simulink model "ControlSystem"  (R2021b)
settings: Solver=VariableStepAuto  StartTime=simIn(1,1)  StopTime=simIn(end,1)  RelTol=1e-3
values from neighbouring files (symbols this model uses):
  A = -inv(L)*R    [PlasmalessModel.m]
  B = L\S    [PlasmalessModel.m]
  C = eye(circuitNumber,length(A))    [PlasmalessModel.m]
  Controller = struct('R1',pid(Rcontr(1,1)),'R2',pid(Rcontr(2,2)),'R3',pid(Rcontr(3,3)),'R4',pid(Rcontr(4,4)),'R5',      pid(Rcontr(5,5)),'R6',pid(Rcontr(6,6)),'R7',pid(Rcontr(7,7)),'R8',pid(Rcontr(8,8)),'R9',pid(Rcontr(9,9)),'R10',      pid(Rcontr(10,10)),'R11',pid(Rcontr(11,11)),'R12',pid(Rcontr(12,12)))    [GeneticAlgorithm.m]    (also in OptimalTunedGA.mat = ; PIDController.m = struct('R1',R1,'R2',R2,'R3',R3,'R4',R4,'R5',R5,'R6',R6,     ; RLocusController.m = struct('R1',R1,'R2',R2,'R3',R3,'R4',R4,'R5',R5,'R6',R6,     )
  D = zeros(circuitNumber,circuitNumber)    [PlasmalessModel.m]
  dt = 0.001    [GeneticAlgorithm.m]    (also in PlasmalessModel.m; ReferenceDatabase.m)
  fil1 = zpk(minreal(R1 - k1 - r1(end)/s, 1e-2))    [RLocusController.m]
  fil10 = zpk(minreal(R10 - k10 - r10(end)/s, 1e-2))    [RLocusController.m]
  fil11 = zpk(minreal(R11 - k11 - r11(end)/s, 1e-2))    [RLocusController.m]
  fil12 = zpk(minreal(R12 - k12 - r12(end)/s, 1e-2))    [RLocusController.m]
  fil2 = zpk(minreal(R2 - k2 - r2(end)/s, 1e-2))    [RLocusController.m]
  fil3 = zpk(minreal(R3 - k3 - r3(end)/s, 1e-2))    [RLocusController.m]
  fil4 = zpk(minreal(R4 - k4 - r4(end)/s, 1e-2))    [RLocusController.m]
  fil5 = zpk(minreal(R5 - k5 - r5(end)/s, 1e-2))    [RLocusController.m]
  fil6 = zpk(minreal(R6 - k6 - r6(end)/s, 1e-2))    [RLocusController.m]
  fil7 = zpk(minreal(R7 - k7 - r7(end)/s, 1e-2))    [RLocusController.m]
  fil8 = zpk(minreal(R8 - k8 - r8(end)/s, 1e-2))    [RLocusController.m]
  fil9 = zpk(minreal(R9 - k9 - r9(end)/s, 1e-2))    [RLocusController.m]
  PSdelay = 1.67e-3    (= 0.00167)    [PlasmalessModel.m]
  PSden = [7e-3 1]    [PlasmalessModel.m]
  PSnum = 1    [PlasmalessModel.m]
  PSsat = [350 350 350 350 350 350           800 800 400 400 330 330]    [PlasmalessModel.m]
  sys1 = balred(sys(1,1),ord)    [PlasmalessModel.m]
  sys10 = balred(sys(10,10),ord)    [PlasmalessModel.m]
  sys11 = balred(sys(11,11),ord)    [PlasmalessModel.m]
  sys12 = balred(sys(12,12),ord)    [PlasmalessModel.m]
  sys2 = balred(sys(2,2),ord)    [PlasmalessModel.m]
  sys3 = balred(sys(3,3),ord)    [PlasmalessModel.m]
  sys4 = balred(sys(4,4),ord)    [PlasmalessModel.m]
  sys5 = balred(sys(5,5),ord)    [PlasmalessModel.m]
  sys6 = balred(sys(6,6),ord)    [PlasmalessModel.m]
  sys7 = balred(sys(7,7),ord)    [PlasmalessModel.m]
  sys8 = balred(sys(8,8),ord)    [PlasmalessModel.m]
  sys9 = balred(sys(9,9),ord)    [PlasmalessModel.m]
  varIpf = Scenario.Reference4.var    [PlasmalessModel.m]    (also in ReferenceDatabase.m)
undefined symbols (not defined in the file or in its folder): k1, k10, k11, k12, k2, k3, k4, k5, k6, k7, k8, k9
libraries: simulink x98, cstblocks x60
(part 3 of 4)

== system ControlSystem/Variant system/SISO/Variant Controller/PID/Subsystem13 ==
  e : Inport
  antiw : Inport  Port=2
  Avoid windup : Constant  Value=0
  Clamping : Subsystem
  Derivative Gain : Gain  Gain=Kd
  Filtered Derivative : TransferFcn  Denominator=Tf
  Integral Gain : Gain  Gain=Ki
  Integrator : Integrator
  Proportional Gain : Gain  Gain=Kp
  Sum action : Sum  Inputs=+++
  Switch1 : Switch  Criteria=u2 > Threshold
  u : Outport
  wires:
  Filtered Derivative/1 -> Sum action/2
  Sum action/1 -> Clamping/1(u), u/1  "u"
  Derivative Gain/1 -> Filtered Derivative/1
  e/1 -> Proportional Gain/1, Clamping/3(e), Integral Gain/1, Derivative Gain/1  "e"
  Switch1/1 -> Integrator/1
  Integral Gain/1 -> Switch1/3
  Avoid windup/1 -> Switch1/1
  Proportional Gain/1 -> Sum action/1
  Integrator/1 -> Sum action/3
  antiw/1 -> Clamping/2(antiw)  "antiw"
  Clamping/1(Clamping) -> Switch1/2  "Clamping"

== system ControlSystem/Variant system/SISO/Variant Controller/PID/Subsystem2 ==
  e : Inport
  antiw : Inport  Port=2
  Avoid windup : Constant  Value=0
  Clamping : Subsystem
  Derivative Gain : Gain  Gain=Kd
  Filtered Derivative : TransferFcn  Denominator=Tf
  Integral Gain : Gain  Gain=Ki
  Integrator : Integrator
  Proportional Gain : Gain  Gain=Kp
  Sum action : Sum  Inputs=+++
  Switch1 : Switch  Criteria=u2 > Threshold
  u : Outport
  wires:
  Clamping/1(Clamping) -> Switch1/2  "Clamping"
  antiw/1 -> Clamping/2(antiw)  "antiw"
  Integrator/1 -> Sum action/3
  Proportional Gain/1 -> Sum action/1
  Avoid windup/1 -> Switch1/1
  Integral Gain/1 -> Switch1/3
  Switch1/1 -> Integrator/1
  e/1 -> Derivative Gain/1, Integral Gain/1, Clamping/3(e), Proportional Gain/1  "e"
  Derivative Gain/1 -> Filtered Derivative/1
  Sum action/1 -> u/1, Clamping/1(u)  "u"
  Filtered Derivative/1 -> Sum action/2

== system ControlSystem/Variant system/SISO/Variant Controller/PID/Subsystem3 ==
  e : Inport
  antiw : Inport  Port=2
  Avoid windup : Constant  Value=0
  Clamping : Subsystem
  Derivative Gain : Gain  Gain=Kd
  Filtered Derivative : TransferFcn  Denominator=Tf
  Integral Gain : Gain  Gain=Ki
  Integrator : Integrator
  Proportional Gain : Gain  Gain=Kp
  Sum action : Sum  Inputs=+++
  Switch1 : Switch  Criteria=u2 > Threshold
  u : Outport
  wires:
  Filtered Derivative/1 -> Sum action/2
  Sum action/1 -> Clamping/1(u), u/1  "u"
  Derivative Gain/1 -> Filtered Derivative/1
  e/1 -> Proportional Gain/1, Clamping/3(e), Integral Gain/1, Derivative Gain/1  "e"
  Switch1/1 -> Integrator/1
  Integral Gain/1 -> Switch1/3
  Avoid windup/1 -> Switch1/1
  Proportional Gain/1 -> Sum action/1
  Integrator/1 -> Sum action/3
  antiw/1 -> Clamping/2(antiw)  "antiw"
  Clamping/1(Clamping) -> Switch1/2  "Clamping"

== system ControlSystem/Variant system/SISO/Variant Controller/PID/Subsystem4 ==
  e : Inport
  antiw : Inport  Port=2
  Avoid windup : Constant  Value=0
  Clamping : Subsystem
  Derivative Gain : Gain  Gain=Kd
  Filtered Derivative : TransferFcn  Denominator=Tf
  Integral Gain : Gain  Gain=Ki
  Integrator : Integrator
  Proportional Gain : Gain  Gain=Kp
  Sum action : Sum  Inputs=+++
  Switch1 : Switch  Criteria=u2 > Threshold
  u : Outport
  wires:
  Clamping/1(Clamping) -> Switch1/2  "Clamping"
  antiw/1 -> Clamping/2(antiw)  "antiw"
  Integrator/1 -> Sum action/3
  Proportional Gain/1 -> Sum action/1
  Avoid windup/1 -> Switch1/1
  Integral Gain/1 -> Switch1/3
  Switch1/1 -> Integrator/1
  e/1 -> Derivative Gain/1, Integral Gain/1, Clamping/3(e), Proportional Gain/1  "e"
  Derivative Gain/1 -> Filtered Derivative/1
  Sum action/1 -> u/1, Clamping/1(u)  "u"
  Filtered Derivative/1 -> Sum action/2

== system ControlSystem/Variant system/SISO/Variant Controller/PID/Subsystem5 ==
  e : Inport
  antiw : Inport  Port=2
  Avoid windup : Constant  Value=0
  Clamping : Subsystem
  Derivative Gain : Gain  Gain=Kd
  Filtered Derivative : TransferFcn  Denominator=Tf
  Integral Gain : Gain  Gain=Ki
  Integrator : Integrator
  Proportional Gain : Gain  Gain=Kp
  Sum action : Sum  Inputs=+++
  Switch1 : Switch  Criteria=u2 > Threshold
  u : Outport
  wires:
  Filtered Derivative/1 -> Sum action/2
  Sum action/1 -> Clamping/1(u), u/1  "u"
  Derivative Gain/1 -> Filtered Derivative/1
  e/1 -> Proportional Gain/1, Clamping/3(e), Integral Gain/1, Derivative Gain/1  "e"
  Switch1/1 -> Integrator/1
  Integral Gain/1 -> Switch1/3
  Avoid windup/1 -> Switch1/1
  Proportional Gain/1 -> Sum action/1
  Integrator/1 -> Sum action/3
  antiw/1 -> Clamping/2(antiw)  "antiw"
  Clamping/1(Clamping) -> Switch1/2  "Clamping"

== system ControlSystem/Variant system/SISO/Variant Controller/PID/Subsystem6 ==
  e : Inport
  antiw : Inport  Port=2
  Avoid windup : Constant  Value=0
  Clamping : Subsystem
  Derivative Gain : Gain  Gain=Kd
  Filtered Derivative : TransferFcn  Denominator=Tf
  Integral Gain : Gain  Gain=Ki
  Integrator : Integrator
  Proportional Gain : Gain  Gain=Kp
  Sum action : Sum  Inputs=+++
  Switch1 : Switch  Criteria=u2 > Threshold
  u : Outport
  wires:
  Clamping/1(Clamping) -> Switch1/2  "Clamping"
  antiw/1 -> Clamping/2(antiw)  "antiw"
  Integrator/1 -> Sum action/3
  Proportional Gain/1 -> Sum action/1
  Avoid windup/1 -> Switch1/1
  Integral Gain/1 -> Switch1/3
  Switch1/1 -> Integrator/1
  e/1 -> Derivative Gain/1, Integral Gain/1, Clamping/3(e), Proportional Gain/1  "e"
  Derivative Gain/1 -> Filtered Derivative/1
  Sum action/1 -> u/1, Clamping/1(u)  "u"
  Filtered Derivative/1 -> Sum action/2

== system ControlSystem/Variant system/SISO/Variant Controller/PID/Subsystem7 ==
  e : Inport
  antiw : Inport  Port=2
  Avoid windup : Constant  Value=0
  Clamping : Subsystem
  Derivative Gain : Gain  Gain=Kd
  Filtered Derivative : TransferFcn  Denominator=Tf
  Integral Gain : Gain  Gain=Ki
  Integrator : Integrator
  Proportional Gain : Gain  Gain=Kp
  Sum action : Sum  Inputs=+++
  Switch1 : Switch  Criteria=u2 > Threshold
  u : Outport
  wires:
  Filtered Derivative/1 -> Sum action/2
  Sum action/1 -> Clamping/1(u), u/1  "u"
  Derivative Gain/1 -> Filtered Derivative/1
  e/1 -> Proportional Gain/1, Clamping/3(e), Integral Gain/1, Derivative Gain/1  "e"
  Switch1/1 -> Integrator/1
  Integral Gain/1 -> Switch1/3
  Avoid windup/1 -> Switch1/1
  Proportional Gain/1 -> Sum action/1
  Integrator/1 -> Sum action/3
  antiw/1 -> Clamping/2(antiw)  "antiw"
  Clamping/1(Clamping) -> Switch1/2  "Clamping"

== system ControlSystem/Variant system/SISO/Variant Controller/PID/Subsystem8 ==
  e : Inport
  antiw : Inport  Port=2
  Avoid windup : Constant  Value=0
  Clamping : Subsystem
  Derivative Gain : Gain  Gain=Kd
  Filtered Derivative : TransferFcn  Denominator=Tf
  Integral Gain : Gain  Gain=Ki
  Integrator : Integrator
  Proportional Gain : Gain  Gain=Kp
  Sum action : Sum  Inputs=+++
  Switch1 : Switch  Criteria=u2 > Threshold
  u : Outport
  wires:
  Clamping/1(Clamping) -> Switch1/2  "Clamping"
  antiw/1 -> Clamping/2(antiw)  "antiw"
  Integrator/1 -> Sum action/3
  Proportional Gain/1 -> Sum action/1
  Avoid windup/1 -> Switch1/1
  Integral Gain/1 -> Switch1/3
  Switch1/1 -> Integrator/1
  e/1 -> Derivative Gain/1, Integral Gain/1, Clamping/3(e), Proportional Gain/1  "e"
  Derivative Gain/1 -> Filtered Derivative/1
  Sum action/1 -> u/1, Clamping/1(u)  "u"
  Filtered Derivative/1 -> Sum action/2

== system ControlSystem/Variant system/SISO/Variant Controller/PID/Subsystem9 ==
  e : Inport
  antiw : Inport  Port=2
  Avoid windup : Constant  Value=0
  Clamping : Subsystem
  Derivative Gain : Gain  Gain=Kd
  Filtered Derivative : TransferFcn  Denominator=Tf
  Integral Gain : Gain  Gain=Ki
  Integrator : Integrator
  Proportional Gain : Gain  Gain=Kp
  Sum action : Sum  Inputs=+++
  Switch1 : Switch  Criteria=u2 > Threshold
  u : Outport
  wires:
  Filtered Derivative/1 -> Sum action/2
  Sum action/1 -> Clamping/1(u), u/1  "u"
  Derivative Gain/1 -> Filtered Derivative/1
  e/1 -> Proportional Gain/1, Clamping/3(e), Integral Gain/1, Derivative Gain/1  "e"
  Switch1/1 -> Integrator/1
  Integral Gain/1 -> Switch1/3
  Avoid windup/1 -> Switch1/1
  Proportional Gain/1 -> Sum action/1
  Integrator/1 -> Sum action/3
  antiw/1 -> Clamping/2(antiw)  "antiw"
  Clamping/1(Clamping) -> Switch1/2  "Clamping"

== system ControlSystem/Variant system/SISO/Variant Controller/Rlocusantiwindup/Subsystem1 ==
  e : Inport
  antiw : Inport  Port=2
  Avoid windup : Constant  Value=0
  Clamping : Subsystem
  Integral Gain : Gain  Gain=Ki
  Integrator : Integrator
  Proportional Gain : Gain  Gain=Kp
  Sum action : Sum  Inputs=+++
  Switch1 : Switch  Criteria=u2 > Threshold
  ZPK compensator : cstblocks/LTI System  sys=Compensator  IC=[]
  u : Outport
  wires:
  Sum action/1 -> Clamping/1(u), u/1  "u"
  ZPK compensator/1 -> Sum action/2
  e/1 -> ZPK compensator/1, Proportional Gain/1, Clamping/3(e), Integral Gain/1  "e"
  Switch1/1 -> Integrator/1
  Integral Gain/1 -> Switch1/3
  Avoid windup/1 -> Switch1/1
  Proportional Gain/1 -> Sum action/1
  Integrator/1 -> Sum action/3
  antiw/1 -> Clamping/2(antiw)  "antiw"
  Clamping/1(Clamping) -> Switch1/2  "Clamping"

== system ControlSystem/Variant system/SISO/Variant Controller/Rlocusantiwindup/Subsystem11 ==
  e : Inport
  antiw : Inport  Port=2
  Avoid windup : Constant  Value=0
  Clamping : Subsystem
  Integral Gain : Gain  Gain=Ki
  Integrator : Integrator
  Proportional Gain : Gain  Gain=Kp
  Sum action : Sum  Inputs=+++
  Switch1 : Switch  Criteria=u2 > Threshold
  ZPK compensator : cstblocks/LTI System  sys=Compensator  IC=[]
  u : Outport
  wires:
  Clamping/1(Clamping) -> Switch1/2  "Clamping"
  antiw/1 -> Clamping/2(antiw)  "antiw"
  Integrator/1 -> Sum action/3
  Proportional Gain/1 -> Sum action/1
  Avoid windup/1 -> Switch1/1
  Integral Gain/1 -> Switch1/3
  Switch1/1 -> Integrator/1
  e/1 -> Integral Gain/1, Clamping/3(e), Proportional Gain/1, ZPK compensator/1  "e"
  ZPK compensator/1 -> Sum action/2
  Sum action/1 -> u/1, Clamping/1(u)  "u"

== system ControlSystem/Variant system/SISO/Variant Controller/Rlocusantiwindup/Subsystem12 ==
  e : Inport
  antiw : Inport  Port=2
  Avoid windup : Constant  Value=0
  Clamping : Subsystem
  Integral Gain : Gain  Gain=Ki
  Integrator : Integrator
  Proportional Gain : Gain  Gain=Kp
  Sum action : Sum  Inputs=+++
  Switch1 : Switch  Criteria=u2 > Threshold
  ZPK compensator : cstblocks/LTI System  sys=Compensator  IC=[]
  u : Outport
  wires:
  Clamping/1(Clamping) -> Switch1/2  "Clamping"
  antiw/1 -> Clamping/2(antiw)  "antiw"
  Integrator/1 -> Sum action/3
  Proportional Gain/1 -> Sum action/1
  Avoid windup/1 -> Switch1/1
  Integral Gain/1 -> Switch1/3
  Switch1/1 -> Integrator/1
  e/1 -> Integral Gain/1, Clamping/3(e), Proportional Gain/1, ZPK compensator/1  "e"
  ZPK compensator/1 -> Sum action/2
  Sum action/1 -> u/1, Clamping/1(u)  "u"

== system ControlSystem/Variant system/SISO/Variant Controller/Rlocusantiwindup/Subsystem15 ==
  e : Inport
  antiw : Inport  Port=2
  Avoid windup : Constant  Value=0
  Clamping : Subsystem
  Integral Gain : Gain  Gain=Ki
  Integrator : Integrator
  Proportional Gain : Gain  Gain=Kp
  Sum action : Sum  Inputs=+++
  Switch1 : Switch  Criteria=u2 > Threshold
  ZPK compensator : cstblocks/LTI System  sys=Compensator  IC=[]
  u : Outport
  wires:
  Sum action/1 -> Clamping/1(u), u/1  "u"
  ZPK compensator/1 -> Sum action/2
  e/1 -> ZPK compensator/1, Proportional Gain/1, Clamping/3(e), Integral Gain/1  "e"
  Switch1/1 -> Integrator/1
  Integral Gain/1 -> Switch1/3
  Avoid windup/1 -> Switch1/1
  Proportional Gain/1 -> Sum action/1
  Integrator/1 -> Sum action/3
  antiw/1 -> Clamping/2(antiw)  "antiw"
  Clamping/1(Clamping) -> Switch1/2  "Clamping"

== system ControlSystem/Variant system/SISO/Variant Controller/Rlocusantiwindup/Subsystem2 ==
  e : Inport
  antiw : Inport  Port=2
  Avoid windup : Constant  Value=0
  Clamping : Subsystem
  Integral Gain : Gain  Gain=Ki
  Integrator : Integrator
  Proportional Gain : Gain  Gain=Kp
  Sum action : Sum  Inputs=+++
  Switch1 : Switch  Criteria=u2 > Threshold
  ZPK compensator : cstblocks/LTI System  sys=Compensator  IC=[]
  u : Outport
  wires:
  Sum action/1 -> Clamping/1(u), u/1  "u"
  ZPK compensator/1 -> Sum action/2
  e/1 -> ZPK compensator/1, Proportional Gain/1, Clamping/3(e), Integral Gain/1  "e"
  Switch1/1 -> Integrator/1
  Integral Gain/1 -> Switch1/3
  Avoid windup/1 -> Switch1/1
  Proportional Gain/1 -> Sum action/1
  Integrator/1 -> Sum action/3
  antiw/1 -> Clamping/2(antiw)  "antiw"
  Clamping/1(Clamping) -> Switch1/2  "Clamping"

== system ControlSystem/Variant system/SISO/Variant Controller/Rlocusantiwindup/Subsystem3 ==
  e : Inport
  antiw : Inport  Port=2
  Avoid windup : Constant  Value=0
  Clamping : Subsystem
  Integral Gain : Gain  Gain=Ki
  Integrator : Integrator
  Proportional Gain : Gain  Gain=Kp
  Sum action : Sum  Inputs=+++
  Switch1 : Switch  Criteria=u2 > Threshold
  ZPK compensator : cstblocks/LTI System  sys=Compensator  IC=[]
  u : Outport
  wires:
  Clamping/1(Clamping) -> Switch1/2  "Clamping"
  antiw/1 -> Clamping/2(antiw)  "antiw"
  Integrator/1 -> Sum action/3
  Proportional Gain/1 -> Sum action/1
  Avoid windup/1 -> Switch1/1
  Integral Gain/1 -> Switch1/3
  Switch1/1 -> Integrator/1
  e/1 -> Integral Gain/1, Clamping/3(e), Proportional Gain/1, ZPK compensator/1  "e"
  ZPK compensator/1 -> Sum action/2
  Sum action/1 -> u/1, Clamping/1(u)  "u"

== system ControlSystem/Variant system/SISO/Variant Controller/Rlocusantiwindup/Subsystem4 ==
  e : Inport
  antiw : Inport  Port=2
  Avoid windup : Constant  Value=0
  Clamping : Subsystem
  Integral Gain : Gain  Gain=Ki
  Integrator : Integrator
  Proportional Gain : Gain  Gain=Kp
  Sum action : Sum  Inputs=+++
  Switch1 : Switch  Criteria=u2 > Threshold
  ZPK compensator : cstblocks/LTI System  sys=Compensator  IC=[]
  u : Outport
  wires:
  Sum action/1 -> Clamping/1(u), u/1  "u"
  ZPK compensator/1 -> Sum action/2
  e/1 -> ZPK compensator/1, Proportional Gain/1, Clamping/3(e), Integral Gain/1  "e"
  Switch1/1 -> Integrator/1
  Integral Gain/1 -> Switch1/3
  Avoid windup/1 -> Switch1/1
  Proportional Gain/1 -> Sum action/1
  Integrator/1 -> Sum action/3
  antiw/1 -> Clamping/2(antiw)  "antiw"
  Clamping/1(Clamping) -> Switch1/2  "Clamping"

== system ControlSystem/Variant system/SISO/Variant Controller/Rlocusantiwindup/Subsystem5 ==
  e : Inport
  antiw : Inport  Port=2
  Avoid windup : Constant  Value=0
  Clamping : Subsystem
  Integral Gain : Gain  Gain=Ki
  Integrator : Integrator
  Proportional Gain : Gain  Gain=Kp
  Sum action : Sum  Inputs=+++
  Switch1 : Switch  Criteria=u2 > Threshold
  ZPK compensator : cstblocks/LTI System  sys=Compensator  IC=[]
  u : Outport
  wires:
  Clamping/1(Clamping) -> Switch1/2  "Clamping"
  antiw/1 -> Clamping/2(antiw)  "antiw"
  Integrator/1 -> Sum action/3
  Proportional Gain/1 -> Sum action/1
  Avoid windup/1 -> Switch1/1
  Integral Gain/1 -> Switch1/3
  Switch1/1 -> Integrator/1
  e/1 -> Integral Gain/1, Clamping/3(e), Proportional Gain/1, ZPK compensator/1  "e"
  ZPK compensator/1 -> Sum action/2
  Sum action/1 -> u/1, Clamping/1(u)  "u"

== system ControlSystem/Variant system/SISO/Variant Controller/Rlocusantiwindup/Subsystem6 ==
  e : Inport
  antiw : Inport  Port=2
  Avoid windup : Constant  Value=0
  Clamping : Subsystem
  Integral Gain : Gain  Gain=Ki
  Integrator : Integrator
  Proportional Gain : Gain  Gain=Kp
  Sum action : Sum  Inputs=+++
  Switch1 : Switch  Criteria=u2 > Threshold
  ZPK compensator : cstblocks/LTI System  sys=Compensator  IC=[]
  u : Outport
  wires:
  Sum action/1 -> Clamping/1(u), u/1  "u"
  ZPK compensator/1 -> Sum action/2
  e/1 -> ZPK compensator/1, Proportional Gain/1, Clamping/3(e), Integral Gain/1  "e"
  Switch1/1 -> Integrator/1
  Integral Gain/1 -> Switch1/3
  Avoid windup/1 -> Switch1/1
  Proportional Gain/1 -> Sum action/1
  Integrator/1 -> Sum action/3
  antiw/1 -> Clamping/2(antiw)  "antiw"
  Clamping/1(Clamping) -> Switch1/2  "Clamping"

== system ControlSystem/Variant system/SISO/Variant Controller/Rlocusantiwindup/Subsystem7 ==
  e : Inport
  antiw : Inport  Port=2
  Avoid windup : Constant  Value=0
  Clamping : Subsystem
  Integral Gain : Gain  Gain=Ki
  Integrator : Integrator
  Proportional Gain : Gain  Gain=Kp
  Sum action : Sum  Inputs=+++
  Switch1 : Switch  Criteria=u2 > Threshold
  ZPK compensator : cstblocks/LTI System  sys=Compensator  IC=[]
  u : Outport
  wires:
  Clamping/1(Clamping) -> Switch1/2  "Clamping"
  antiw/1 -> Clamping/2(antiw)  "antiw"
  Integrator/1 -> Sum action/3
  Proportional Gain/1 -> Sum action/1
  Avoid windup/1 -> Switch1/1
  Integral Gain/1 -> Switch1/3
  Switch1/1 -> Integrator/1
  e/1 -> Integral Gain/1, Clamping/3(e), Proportional Gain/1, ZPK compensator/1  "e"
  ZPK compensator/1 -> Sum action/2
  Sum action/1 -> u/1, Clamping/1(u)  "u"

== system ControlSystem/Variant system/SISO/Variant Controller/Rlocusantiwindup/Subsystem8 ==
  e : Inport
  antiw : Inport  Port=2
  Avoid windup : Constant  Value=0
  Clamping : Subsystem
  Integral Gain : Gain  Gain=Ki
  Integrator : Integrator
  Proportional Gain : Gain  Gain=Kp
  Sum action : Sum  Inputs=+++
  Switch1 : Switch  Criteria=u2 > Threshold
  ZPK compensator : cstblocks/LTI System  sys=Compensator  IC=[]
  u : Outport
  wires:
  Sum action/1 -> Clamping/1(u), u/1  "u"
  ZPK compensator/1 -> Sum action/2
  e/1 -> ZPK compensator/1, Proportional Gain/1, Clamping/3(e), Integral Gain/1  "e"
  Switch1/1 -> Integrator/1
  Integral Gain/1 -> Switch1/3
  Avoid windup/1 -> Switch1/1
  Proportional Gain/1 -> Sum action/1
  Integrator/1 -> Sum action/3
  antiw/1 -> Clamping/2(antiw)  "antiw"
  Clamping/1(Clamping) -> Switch1/2  "Clamping"

== system ControlSystem/Variant system/SISO/Variant Controller/Rlocusantiwindup/Subsystem9 ==
  e : Inport
  antiw : Inport  Port=2
  Avoid windup : Constant  Value=0
  Clamping : Subsystem
  Integral Gain : Gain  Gain=Ki
  Integrator : Integrator
  Proportional Gain : Gain  Gain=Kp
  Sum action : Sum  Inputs=+++
  Switch1 : Switch  Criteria=u2 > Threshold
  ZPK compensator : cstblocks/LTI System  sys=Compensator  IC=[]
  u : Outport
  wires:
  Clamping/1(Clamping) -> Switch1/2  "Clamping"
  antiw/1 -> Clamping/2(antiw)  "antiw"
  Integrator/1 -> Sum action/3
  Proportional Gain/1 -> Sum action/1
  Avoid windup/1 -> Switch1/1
  Integral Gain/1 -> Switch1/3
  Switch1/1 -> Integrator/1
  e/1 -> Integral Gain/1, Clamping/3(e), Proportional Gain/1, ZPK compensator/1  "e"
  ZPK compensator/1 -> Sum action/2
  Sum action/1 -> u/1, Clamping/1(u)  "u"

== system ControlSystem/Variant system/MIMO/Variant Controller/PID/Subsystem1/Clamping ==
  u : Inport
  antiw : Inport  Port=2
  e : Inport  Port=3
  Abs : Abs
  Compare To Threshold : simulink/Logic and Bit Operations/Compare To Constant  relop=>=  const=Threshold  OutDataTypeStr=boolean
  Compare To Zero : simulink/Logic and Bit Operations/Compare To Zero  relop=>  OutDataTypeStr=boolean
  Logical Operator : Logic  OutDataTypeStr=boolean
  Product : Product
  Clamping : Outport
  wires:
  u/1 -> Product/2
  Logical Operator/1 -> Clamping/1  "Clamping"
  e/1 -> Product/1
  Abs/1 -> Compare To Threshold/1
  Product/1 -> Compare To Zero/1
  Compare To Threshold/1 -> Logical Operator/1
  Compare To Zero/1 -> Logical Operator/2
  antiw/1 -> Abs/1

== system ControlSystem/Variant system/MIMO/Variant Controller/PID/Subsystem10/Clamping ==
  u : Inport
  antiw : Inport  Port=2
  e : Inport  Port=3
  Abs : Abs
  Compare To Threshold : simulink/Logic and Bit Operations/Compare To Constant  relop=>=  const=Threshold  OutDataTypeStr=boolean
  Compare To Zero : simulink/Logic and Bit Operations/Compare To Zero  relop=>  OutDataTypeStr=boolean
  Logical Operator : Logic  OutDataTypeStr=boolean
  Product : Product
  Clamping : Outport
  wires:
  u/1 -> Product/2
  Logical Operator/1 -> Clamping/1  "Clamping"
  e/1 -> Product/1
  Abs/1 -> Compare To Threshold/1
  Product/1 -> Compare To Zero/1
  Compare To Threshold/1 -> Logical Operator/1
  Compare To Zero/1 -> Logical Operator/2
  antiw/1 -> Abs/1

== system ControlSystem/Variant system/MIMO/Variant Controller/PID/Subsystem11/Clamping ==
  u : Inport
  antiw : Inport  Port=2
  e : Inport  Port=3
  Abs : Abs
  Compare To Threshold : simulink/Logic and Bit Operations/Compare To Constant  relop=>=  const=Threshold  OutDataTypeStr=boolean
  Compare To Zero : simulink/Logic and Bit Operations/Compare To Zero  relop=>  OutDataTypeStr=boolean
  Logical Operator : Logic  OutDataTypeStr=boolean
  Product : Product
  Clamping : Outport
  wires:
  antiw/1 -> Abs/1
  Compare To Zero/1 -> Logical Operator/2
  Compare To Threshold/1 -> Logical Operator/1
  Product/1 -> Compare To Zero/1
  Abs/1 -> Compare To Threshold/1
  e/1 -> Product/1
  Logical Operator/1 -> Clamping/1  "Clamping"
  u/1 -> Product/2

== system ControlSystem/Variant system/MIMO/Variant Controller/PID/Subsystem13/Clamping ==
  u : Inport
  antiw : Inport  Port=2
  e : Inport  Port=3
  Abs : Abs
  Compare To Threshold : simulink/Logic and Bit Operations/Compare To Constant  relop=>=  const=Threshold  OutDataTypeStr=boolean
  Compare To Zero : simulink/Logic and Bit Operations/Compare To Zero  relop=>  OutDataTypeStr=boolean
  Logical Operator : Logic  OutDataTypeStr=boolean
  Product : Product
  Clamping : Outport
  wires:
  antiw/1 -> Abs/1
  Compare To Zero/1 -> Logical Operator/2
  Compare To Threshold/1 -> Logical Operator/1
  Product/1 -> Compare To Zero/1
  Abs/1 -> Compare To Threshold/1
  e/1 -> Product/1
  Logical Operator/1 -> Clamping/1  "Clamping"
  u/1 -> Product/2

== system ControlSystem/Variant system/MIMO/Variant Controller/PID/Subsystem2/Clamping ==
  u : Inport
  antiw : Inport  Port=2
  e : Inport  Port=3
  Abs : Abs
  Compare To Threshold : simulink/Logic and Bit Operations/Compare To Constant  relop=>=  const=Threshold  OutDataTypeStr=boolean
  Compare To Zero : simulink/Logic and Bit Operations/Compare To Zero  relop=>  OutDataTypeStr=boolean
  Logical Operator : Logic  OutDataTypeStr=boolean
  Product : Product
  Clamping : Outport
  wires:
  u/1 -> Product/2
  Logical Operator/1 -> Clamping/1  "Clamping"
  e/1 -> Product/1
  Abs/1 -> Compare To Threshold/1
  Product/1 -> Compare To Zero/1
  Compare To Threshold/1 -> Logical Operator/1
  Compare To Zero/1 -> Logical Operator/2
  antiw/1 -> Abs/1

== system ControlSystem/Variant system/MIMO/Variant Controller/PID/Subsystem3/Clamping ==
  u : Inport
  antiw : Inport  Port=2
  e : Inport  Port=3
  Abs : Abs
  Compare To Threshold : simulink/Logic and Bit Operations/Compare To Constant  relop=>=  const=Threshold  OutDataTypeStr=boolean
  Compare To Zero : simulink/Logic and Bit Operations/Compare To Zero  relop=>  OutDataTypeStr=boolean
  Logical Operator : Logic  OutDataTypeStr=boolean
  Product : Product
  Clamping : Outport
  wires:
  antiw/1 -> Abs/1
  Compare To Zero/1 -> Logical Operator/2
  Compare To Threshold/1 -> Logical Operator/1
  Product/1 -> Compare To Zero/1
  Abs/1 -> Compare To Threshold/1
  e/1 -> Product/1
  Logical Operator/1 -> Clamping/1  "Clamping"
  u/1 -> Product/2

== system ControlSystem/Variant system/MIMO/Variant Controller/PID/Subsystem4/Clamping ==
  u : Inport
  antiw : Inport  Port=2
  e : Inport  Port=3
  Abs : Abs
  Compare To Threshold : simulink/Logic and Bit Operations/Compare To Constant  relop=>=  const=Threshold  OutDataTypeStr=boolean
  Compare To Zero : simulink/Logic and Bit Operations/Compare To Zero  relop=>  OutDataTypeStr=boolean
  Logical Operator : Logic  OutDataTypeStr=boolean
  Product : Product
  Clamping : Outport
  wires:
  u/1 -> Product/2
  Logical Operator/1 -> Clamping/1  "Clamping"
  e/1 -> Product/1
  Abs/1 -> Compare To Threshold/1
  Product/1 -> Compare To Zero/1
  Compare To Threshold/1 -> Logical Operator/1
  Compare To Zero/1 -> Logical Operator/2
  antiw/1 -> Abs/1

== system ControlSystem/Variant system/MIMO/Variant Controller/PID/Subsystem5/Clamping ==
  u : Inport
  antiw : Inport  Port=2
  e : Inport  Port=3
  Abs : Abs
  Compare To Threshold : simulink/Logic and Bit Operations/Compare To Constant  relop=>=  const=Threshold  OutDataTypeStr=boolean
  Compare To Zero : simulink/Logic and Bit Operations/Compare To Zero  relop=>  OutDataTypeStr=boolean
  Logical Operator : Logic  OutDataTypeStr=boolean
  Product : Product
  Clamping : Outport
  wires:
  antiw/1 -> Abs/1
  Compare To Zero/1 -> Logical Operator/2
  Compare To Threshold/1 -> Logical Operator/1
  Product/1 -> Compare To Zero/1
  Abs/1 -> Compare To Threshold/1
  e/1 -> Product/1
  Logical Operator/1 -> Clamping/1  "Clamping"
  u/1 -> Product/2

== system ControlSystem/Variant system/MIMO/Variant Controller/PID/Subsystem6/Clamping ==
  u : Inport
  antiw : Inport  Port=2
  e : Inport  Port=3
  Abs : Abs
  Compare To Threshold : simulink/Logic and Bit Operations/Compare To Constant  relop=>=  const=Threshold  OutDataTypeStr=boolean
  Compare To Zero : simulink/Logic and Bit Operations/Compare To Zero  relop=>  OutDataTypeStr=boolean
  Logical Operator : Logic  OutDataTypeStr=boolean
  Product : Product
  Clamping : Outport
  wires:
  u/1 -> Product/2
  Logical Operator/1 -> Clamping/1  "Clamping"
  e/1 -> Product/1
  Abs/1 -> Compare To Threshold/1
  Product/1 -> Compare To Zero/1
  Compare To Threshold/1 -> Logical Operator/1
  Compare To Zero/1 -> Logical Operator/2
  antiw/1 -> Abs/1

== system ControlSystem/Variant system/MIMO/Variant Controller/PID/Subsystem7/Clamping ==
  u : Inport
  antiw : Inport  Port=2
  e : Inport  Port=3
  Abs : Abs
  Compare To Threshold : simulink/Logic and Bit Operations/Compare To Constant  relop=>=  const=Threshold  OutDataTypeStr=boolean
  Compare To Zero : simulink/Logic and Bit Operations/Compare To Zero  relop=>  OutDataTypeStr=boolean
  Logical Operator : Logic  OutDataTypeStr=boolean
  Product : Product
  Clamping : Outport
  wires:
  antiw/1 -> Abs/1
  Compare To Zero/1 -> Logical Operator/2
  Compare To Threshold/1 -> Logical Operator/1
  Product/1 -> Compare To Zero/1
  Abs/1 -> Compare To Threshold/1
  e/1 -> Product/1
  Logical Operator/1 -> Clamping/1  "Clamping"
  u/1 -> Product/2

== system ControlSystem/Variant system/MIMO/Variant Controller/PID/Subsystem8/Clamping ==
  u : Inport
  antiw : Inport  Port=2
  e : Inport  Port=3
  Abs : Abs
  Compare To Threshold : simulink/Logic and Bit Operations/Compare To Constant  relop=>=  const=Threshold  OutDataTypeStr=boolean
  Compare To Zero : simulink/Logic and Bit Operations/Compare To Zero  relop=>  OutDataTypeStr=boolean
  Logical Operator : Logic  OutDataTypeStr=boolean
  Product : Product
  Clamping : Outport
  wires:
  u/1 -> Product/2
  Logical Operator/1 -> Clamping/1  "Clamping"
  e/1 -> Product/1
  Abs/1 -> Compare To Threshold/1
  Product/1 -> Compare To Zero/1
  Compare To Threshold/1 -> Logical Operator/1
  Compare To Zero/1 -> Logical Operator/2
  antiw/1 -> Abs/1

== system ControlSystem/Variant system/MIMO/Variant Controller/PID/Subsystem9/Clamping ==
  u : Inport
  antiw : Inport  Port=2
  e : Inport  Port=3
  Abs : Abs
  Compare To Threshold : simulink/Logic and Bit Operations/Compare To Constant  relop=>=  const=Threshold  OutDataTypeStr=boolean
  Compare To Zero : simulink/Logic and Bit Operations/Compare To Zero  relop=>  OutDataTypeStr=boolean
  Logical Operator : Logic  OutDataTypeStr=boolean
  Product : Product
  Clamping : Outport
  wires:
  antiw/1 -> Abs/1
  Compare To Zero/1 -> Logical Operator/2
  Compare To Threshold/1 -> Logical Operator/1
  Product/1 -> Compare To Zero/1
  Abs/1 -> Compare To Threshold/1
  e/1 -> Product/1
  Logical Operator/1 -> Clamping/1  "Clamping"
  u/1 -> Product/2

== system ControlSystem/Variant system/MIMO/Variant Controller/Rlocusantiwindup/Subsystem1/Clamping ==
  u : Inport
  antiw : Inport  Port=2
  e : Inport  Port=3
  Abs : Abs
  Compare To Threshold : simulink/Logic and Bit Operations/Compare To Constant  relop=>=  const=Threshold  OutDataTypeStr=boolean
  Compare To Zero : simulink/Logic and Bit Operations/Compare To Zero  relop=>=  OutDataTypeStr=boolean
  Logical Operator : Logic  OutDataTypeStr=boolean
  Product : Product
  Clamping : Outport
  wires:
  antiw/1 -> Abs/1
  Compare To Zero/1 -> Logical Operator/2
  Compare To Threshold/1 -> Logical Operator/1
  Product/1 -> Compare To Zero/1
  Abs/1 -> Compare To Threshold/1
  e/1 -> Product/1
  Logical Operator/1 -> Clamping/1  "Clamping"
  u/1 -> Product/2

== system ControlSystem/Variant system/MIMO/Variant Controller/Rlocusantiwindup/Subsystem11/Clamping ==
  u : Inport
  antiw : Inport  Port=2
  e : Inport  Port=3
  Abs : Abs
  Compare To Threshold : simulink/Logic and Bit Operations/Compare To Constant  relop=>=  const=Threshold  OutDataTypeStr=boolean
  Compare To Zero : simulink/Logic and Bit Operations/Compare To Zero  relop=>=  OutDataTypeStr=boolean
  Logical Operator : Logic  OutDataTypeStr=boolean
  Product : Product
  Clamping : Outport
  wires:
  u/1 -> Product/2
  Logical Operator/1 -> Clamping/1  "Clamping"
  e/1 -> Product/1
  Abs/1 -> Compare To Threshold/1
  Product/1 -> Compare To Zero/1
  Compare To Threshold/1 -> Logical Operator/1
  Compare To Zero/1 -> Logical Operator/2
  antiw/1 -> Abs/1

== system ControlSystem/Variant system/MIMO/Variant Controller/Rlocusantiwindup/Subsystem12/Clamping ==
  u : Inport
  antiw : Inport  Port=2
  e : Inport  Port=3
  Abs : Abs
  Compare To Threshold : simulink/Logic and Bit Operations/Compare To Constant  relop=>=  const=Threshold  OutDataTypeStr=boolean
  Compare To Zero : simulink/Logic and Bit Operations/Compare To Zero  relop=>=  OutDataTypeStr=boolean
  Logical Operator : Logic  OutDataTypeStr=boolean
  Product : Product
  Clamping : Outport
  wires:
  u/1 -> Product/2
  Logical Operator/1 -> Clamping/1  "Clamping"
  e/1 -> Product/1
  Abs/1 -> Compare To Threshold/1
  Product/1 -> Compare To Zero/1
  Compare To Threshold/1 -> Logical Operator/1
  Compare To Zero/1 -> Logical Operator/2
  antiw/1 -> Abs/1

== system ControlSystem/Variant system/MIMO/Variant Controller/Rlocusantiwindup/Subsystem15/Clamping ==
  u : Inport
  antiw : Inport  Port=2
  e : Inport  Port=3
  Abs : Abs
  Compare To Threshold : simulink/Logic and Bit Operations/Compare To Constant  relop=>=  const=Threshold  OutDataTypeStr=boolean
  Compare To Zero : simulink/Logic and Bit Operations/Compare To Zero  relop=>=  OutDataTypeStr=boolean
  Logical Operator : Logic  OutDataTypeStr=boolean
  Product : Product
  Clamping : Outport
  wires:
  antiw/1 -> Abs/1
  Compare To Zero/1 -> Logical Operator/2
  Compare To Threshold/1 -> Logical Operator/1
  Product/1 -> Compare To Zero/1
  Abs/1 -> Compare To Threshold/1
  e/1 -> Product/1
  Logical Operator/1 -> Clamping/1  "Clamping"
  u/1 -> Product/2

== system ControlSystem/Variant system/MIMO/Variant Controller/Rlocusantiwindup/Subsystem2/Clamping ==
  u : Inport
  antiw : Inport  Port=2
  e : Inport  Port=3
  Abs : Abs
  Compare To Threshold : simulink/Logic and Bit Operations/Compare To Constant  relop=>=  const=Threshold  OutDataTypeStr=boolean
  Compare To Zero : simulink/Logic and Bit Operations/Compare To Zero  relop=>=  OutDataTypeStr=boolean
  Logical Operator : Logic  OutDataTypeStr=boolean
  Product : Product
  Clamping : Outport
  wires:
  antiw/1 -> Abs/1
  Compare To Zero/1 -> Logical Operator/2
  Compare To Threshold/1 -> Logical Operator/1
  Product/1 -> Compare To Zero/1
  Abs/1 -> Compare To Threshold/1
  e/1 -> Product/1
  Logical Operator/1 -> Clamping/1  "Clamping"
  u/1 -> Product/2

== system ControlSystem/Variant system/MIMO/Variant Controller/Rlocusantiwindup/Subsystem3/Clamping ==
  u : Inport
  antiw : Inport  Port=2
  e : Inport  Port=3
  Abs : Abs
  Compare To Threshold : simulink/Logic and Bit Operations/Compare To Constant  relop=>=  const=Threshold  OutDataTypeStr=boolean
  Compare To Zero : simulink/Logic and Bit Operations/Compare To Zero  relop=>=  OutDataTypeStr=boolean
  Logical Operator : Logic  OutDataTypeStr=boolean
  Product : Product
  Clamping : Outport
  wires:
  u/1 -> Product/2
  Logical Operator/1 -> Clamping/1  "Clamping"
  e/1 -> Product/1
  Abs/1 -> Compare To Threshold/1
  Product/1 -> Compare To Zero/1
  Compare To Threshold/1 -> Logical Operator/1
  Compare To Zero/1 -> Logical Operator/2
  antiw/1 -> Abs/1

== system ControlSystem/Variant system/MIMO/Variant Controller/Rlocusantiwindup/Subsystem4/Clamping ==
  u : Inport
  antiw : Inport  Port=2
  e : Inport  Port=3
  Abs : Abs
  Compare To Threshold : simulink/Logic and Bit Operations/Compare To Constant  relop=>=  const=Threshold  OutDataTypeStr=boolean
  Compare To Zero : simulink/Logic and Bit Operations/Compare To Zero  relop=>=  OutDataTypeStr=boolean
  Logical Operator : Logic  OutDataTypeStr=boolean
  Product : Product
  Clamping : Outport
  wires:
  antiw/1 -> Abs/1
  Compare To Zero/1 -> Logical Operator/2
  Compare To Threshold/1 -> Logical Operator/1
  Product/1 -> Compare To Zero/1
  Abs/1 -> Compare To Threshold/1
  e/1 -> Product/1
  Logical Operator/1 -> Clamping/1  "Clamping"
  u/1 -> Product/2

== system ControlSystem/Variant system/MIMO/Variant Controller/Rlocusantiwindup/Subsystem5/Clamping ==
  u : Inport
  antiw : Inport  Port=2
  e : Inport  Port=3
  Abs : Abs
  Compare To Threshold : simulink/Logic and Bit Operations/Compare To Constant  relop=>=  const=Threshold  OutDataTypeStr=boolean
  Compare To Zero : simulink/Logic and Bit Operations/Compare To Zero  relop=>=  OutDataTypeStr=boolean
  Logical Operator : Logic  OutDataTypeStr=boolean
  Product : Product
  Clamping : Outport
  wires:
  u/1 -> Product/2
  Logical Operator/1 -> Clamping/1  "Clamping"
  e/1 -> Product/1
  Abs/1 -> Compare To Threshold/1
  Product/1 -> Compare To Zero/1
  Compare To Threshold/1 -> Logical Operator/1
  Compare To Zero/1 -> Logical Operator/2
  antiw/1 -> Abs/1

== system ControlSystem/Variant system/MIMO/Variant Controller/Rlocusantiwindup/Subsystem6/Clamping ==
  u : Inport
  antiw : Inport  Port=2
  e : Inport  Port=3
  Abs : Abs
  Compare To Threshold : simulink/Logic and Bit Operations/Compare To Constant  relop=>=  const=Threshold  OutDataTypeStr=boolean
  Compare To Zero : simulink/Logic and Bit Operations/Compare To Zero  relop=>=  OutDataTypeStr=boolean
  Logical Operator : Logic  OutDataTypeStr=boolean
  Product : Product
  Clamping : Outport
  wires:
  antiw/1 -> Abs/1
  Compare To Zero/1 -> Logical Operator/2
  Compare To Threshold/1 -> Logical Operator/1
  Product/1 -> Compare To Zero/1
  Abs/1 -> Compare To Threshold/1
  e/1 -> Product/1
  Logical Operator/1 -> Clamping/1  "Clamping"
  u/1 -> Product/2

== system ControlSystem/Variant system/MIMO/Variant Controller/Rlocusantiwindup/Subsystem7/Clamping ==
  u : Inport
  antiw : Inport  Port=2
  e : Inport  Port=3
  Abs : Abs
  Compare To Threshold : simulink/Logic and Bit Operations/Compare To Constant  relop=>=  const=Threshold  OutDataTypeStr=boolean
  Compare To Zero : simulink/Logic and Bit Operations/Compare To Zero  relop=>=  OutDataTypeStr=boolean
  Logical Operator : Logic  OutDataTypeStr=boolean
  Product : Product
  Clamping : Outport
  wires:
  u/1 -> Product/2
  Logical Operator/1 -> Clamping/1  "Clamping"
  e/1 -> Product/1
  Abs/1 -> Compare To Threshold/1
  Product/1 -> Compare To Zero/1
  Compare To Threshold/1 -> Logical Operator/1
  Compare To Zero/1 -> Logical Operator/2
  antiw/1 -> Abs/1

== system ControlSystem/Variant system/MIMO/Variant Controller/Rlocusantiwindup/Subsystem8/Clamping ==
  u : Inport
  antiw : Inport  Port=2
  e : Inport  Port=3
  Abs : Abs
  Compare To Threshold : simulink/Logic and Bit Operations/Compare To Constant  relop=>=  const=Threshold  OutDataTypeStr=boolean
  Compare To Zero : simulink/Logic and Bit Operations/Compare To Zero  relop=>=  OutDataTypeStr=boolean
  Logical Operator : Logic  OutDataTypeStr=boolean
  Product : Product
  Clamping : Outport
  wires:
  antiw/1 -> Abs/1
  Compare To Zero/1 -> Logical Operator/2
  Compare To Threshold/1 -> Logical Operator/1
  Product/1 -> Compare To Zero/1
  Abs/1 -> Compare To Threshold/1
  e/1 -> Product/1
  Logical Operator/1 -> Clamping/1  "Clamping"
  u/1 -> Product/2

== system ControlSystem/Variant system/MIMO/Variant Controller/Rlocusantiwindup/Subsystem9/Clamping ==
  u : Inport
  antiw : Inport  Port=2
  e : Inport  Port=3
  Abs : Abs
  Compare To Threshold : simulink/Logic and Bit Operations/Compare To Constant  relop=>=  const=Threshold  OutDataTypeStr=boolean
  Compare To Zero : simulink/Logic and Bit Operations/Compare To Zero  relop=>=  OutDataTypeStr=boolean
  Logical Operator : Logic  OutDataTypeStr=boolean
  Product : Product
  Clamping : Outport
  wires:
  u/1 -> Product/2
  Logical Operator/1 -> Clamping/1  "Clamping"
  e/1 -> Product/1
  Abs/1 -> Compare To Threshold/1
  Product/1 -> Compare To Zero/1
  Compare To Threshold/1 -> Logical Operator/1
  Compare To Zero/1 -> Logical Operator/2
  antiw/1 -> Abs/1

== system ControlSystem/Variant system/SISO/Variant Controller/PID/Subsystem1/Clamping ==
  u : Inport
  antiw : Inport  Port=2
  e : Inport  Port=3
  Abs : Abs
  Compare To Threshold : simulink/Logic and Bit Operations/Compare To Constant  relop=>=  const=Threshold  OutDataTypeStr=boolean
  Compare To Zero : simulink/Logic and Bit Operations/Compare To Zero  relop=>=  OutDataTypeStr=boolean
  Logical Operator : Logic  OutDataTypeStr=boolean
  Product : Product
  Clamping : Outport
  wires:
  u/1 -> Product/2
  Logical Operator/1 -> Clamping/1  "Clamping"
  e/1 -> Product/1
  Abs/1 -> Compare To Threshold/1
  Product/1 -> Compare To Zero/1
  Compare To Threshold/1 -> Logical Operator/1
  Compare To Zero/1 -> Logical Operator/2
  antiw/1 -> Abs/1

== system ControlSystem/Variant system/SISO/Variant Controller/PID/Subsystem10/Clamping ==
  u : Inport
  antiw : Inport  Port=2
  e : Inport  Port=3
  Abs : Abs
  Compare To Threshold : simulink/Logic and Bit Operations/Compare To Constant  relop=>=  const=Threshold  OutDataTypeStr=boolean
  Compare To Zero : simulink/Logic and Bit Operations/Compare To Zero  relop=>=  OutDataTypeStr=boolean
  Logical Operator : Logic  OutDataTypeStr=boolean
  Product : Product
  Clamping : Outport
  wires:
  u/1 -> Product/2
  Logical Operator/1 -> Clamping/1  "Clamping"
  e/1 -> Product/1
  Abs/1 -> Compare To Threshold/1
  Product/1 -> Compare To Zero/1
  Compare To Threshold/1 -> Logical Operator/1
  Compare To Zero/1 -> Logical Operator/2
  antiw/1 -> Abs/1

== system ControlSystem/Variant system/SISO/Variant Controller/PID/Subsystem11/Clamping ==
  u : Inport
  antiw : Inport  Port=2
  e : Inport  Port=3
  Abs : Abs
  Compare To Threshold : simulink/Logic and Bit Operations/Compare To Constant  relop=>=  const=Threshold  OutDataTypeStr=boolean
  Compare To Zero : simulink/Logic and Bit Operations/Compare To Zero  relop=>=  OutDataTypeStr=boolean
  Logical Operator : Logic  OutDataTypeStr=boolean
  Product : Product
  Clamping : Outport
  wires:
  antiw/1 -> Abs/1
  Compare To Zero/1 -> Logical Operator/2
  Compare To Threshold/1 -> Logical Operator/1
  Product/1 -> Compare To Zero/1
  Abs/1 -> Compare To Threshold/1
  e/1 -> Product/1
  Logical Operator/1 -> Clamping/1  "Clamping"
  u/1 -> Product/2

== system ControlSystem/Variant system/SISO/Variant Controller/PID/Subsystem13/Clamping ==
  u : Inport
  antiw : Inport  Port=2
  e : Inport  Port=3
  Abs : Abs
  Compare To Threshold : simulink/Logic and Bit Operations/Compare To Constant  relop=>=  const=Threshold  OutDataTypeStr=boolean
  Compare To Zero : simulink/Logic and Bit Operations/Compare To Zero  relop=>=  OutDataTypeStr=boolean
  Logical Operator : Logic  OutDataTypeStr=boolean
  Product : Product
  Clamping : Outport
  wires:
  antiw/1 -> Abs/1
  Compare To Zero/1 -> Logical Operator/2
  Compare To Threshold/1 -> Logical Operator/1
  Product/1 -> Compare To Zero/1
  Abs/1 -> Compare To Threshold/1
  e/1 -> Product/1
  Logical Operator/1 -> Clamping/1  "Clamping"
  u/1 -> Product/2

== system ControlSystem/Variant system/SISO/Variant Controller/PID/Subsystem2/Clamping ==
  u : Inport
  antiw : Inport  Port=2
  e : Inport  Port=3
  Abs : Abs
  Compare To Threshold : simulink/Logic and Bit Operations/Compare To Constant  relop=>=  const=Threshold  OutDataTypeStr=boolean
  Compare To Zero : simulink/Logic and Bit Operations/Compare To Zero  relop=>=  OutDataTypeStr=boolean
  Logical Operator : Logic  OutDataTypeStr=boolean
  Product : Product
  Clamping : Outport
  wires:
  u/1 -> Product/2
  Logical Operator/1 -> Clamping/1  "Clamping"
  e/1 -> Product/1
  Abs/1 -> Compare To Threshold/1
  Product/1 -> Compare To Zero/1
  Compare To Threshold/1 -> Logical Operator/1
  Compare To Zero/1 -> Logical Operator/2
  antiw/1 -> Abs/1

== system ControlSystem/Variant system/SISO/Variant Controller/PID/Subsystem3/Clamping ==
  u : Inport
  antiw : Inport  Port=2
  e : Inport  Port=3
  Abs : Abs
  Compare To Threshold : simulink/Logic and Bit Operations/Compare To Constant  relop=>=  const=Threshold  OutDataTypeStr=boolean
  Compare To Zero : simulink/Logic and Bit Operations/Compare To Zero  relop=>=  OutDataTypeStr=boolean
  Logical Operator : Logic  OutDataTypeStr=boolean
  Product : Product
  Clamping : Outport
  wires:
  antiw/1 -> Abs/1
  Compare To Zero/1 -> Logical Operator/2
  Compare To Threshold/1 -> Logical Operator/1
  Product/1 -> Compare To Zero/1
  Abs/1 -> Compare To Threshold/1
  e/1 -> Product/1
  Logical Operator/1 -> Clamping/1  "Clamping"
  u/1 -> Product/2

== system ControlSystem/Variant system/SISO/Variant Controller/PID/Subsystem4/Clamping ==
  u : Inport
  antiw : Inport  Port=2
  e : Inport  Port=3
  Abs : Abs
  Compare To Threshold : simulink/Logic and Bit Operations/Compare To Constant  relop=>=  const=Threshold  OutDataTypeStr=boolean
  Compare To Zero : simulink/Logic and Bit Operations/Compare To Zero  relop=>=  OutDataTypeStr=boolean
  Logical Operator : Logic  OutDataTypeStr=boolean
  Product : Product
  Clamping : Outport
  wires:
  u/1 -> Product/2
  Logical Operator/1 -> Clamping/1  "Clamping"
  e/1 -> Product/1
  Abs/1 -> Compare To Threshold/1
  Product/1 -> Compare To Zero/1
  Compare To Threshold/1 -> Logical Operator/1
  Compare To Zero/1 -> Logical Operator/2
  antiw/1 -> Abs/1

== system ControlSystem/Variant system/SISO/Variant Controller/PID/Subsystem5/Clamping ==
  u : Inport
  antiw : Inport  Port=2
  e : Inport  Port=3
  Abs : Abs
  Compare To Threshold : simulink/Logic and Bit Operations/Compare To Constant  relop=>=  const=Threshold  OutDataTypeStr=boolean
  Compare To Zero : simulink/Logic and Bit Operations/Compare To Zero  relop=>=  OutDataTypeStr=boolean
  Logical Operator : Logic  OutDataTypeStr=boolean
  Product : Product
  Clamping : Outport
  wires:
  antiw/1 -> Abs/1
  Compare To Zero/1 -> Logical Operator/2
  Compare To Threshold/1 -> Logical Operator/1
  Product/1 -> Compare To Zero/1
  Abs/1 -> Compare To Threshold/1
  e/1 -> Product/1
  Logical Operator/1 -> Clamping/1  "Clamping"
  u/1 -> Product/2

== system ControlSystem/Variant system/SISO/Variant Controller/PID/Subsystem6/Clamping ==
  u : Inport
  antiw : Inport  Port=2
  e : Inport  Port=3
  Abs : Abs
  Compare To Threshold : simulink/Logic and Bit Operations/Compare To Constant  relop=>=  const=Threshold  OutDataTypeStr=boolean
  Compare To Zero : simulink/Logic and Bit Operations/Compare To Zero  relop=>=  OutDataTypeStr=boolean
  Logical Operator : Logic  OutDataTypeStr=boolean
  Product : Product
  Clamping : Outport
  wires:
  u/1 -> Product/2
  Logical Operator/1 -> Clamping/1  "Clamping"
  e/1 -> Product/1
  Abs/1 -> Compare To Threshold/1
  Product/1 -> Compare To Zero/1
  Compare To Threshold/1 -> Logical Operator/1
  Compare To Zero/1 -> Logical Operator/2
  antiw/1 -> Abs/1

== system ControlSystem/Variant system/SISO/Variant Controller/PID/Subsystem7/Clamping ==
  u : Inport
  antiw : Inport  Port=2
  e : Inport  Port=3
  Abs : Abs
  Compare To Threshold : simulink/Logic and Bit Operations/Compare To Constant  relop=>=  const=Threshold  OutDataTypeStr=boolean
  Compare To Zero : simulink/Logic and Bit Operations/Compare To Zero  relop=>=  OutDataTypeStr=boolean
  Logical Operator : Logic  OutDataTypeStr=boolean
  Product : Product
  Clamping : Outport
  wires:
  antiw/1 -> Abs/1
  Compare To Zero/1 -> Logical Operator/2
  Compare To Threshold/1 -> Logical Operator/1
  Product/1 -> Compare To Zero/1
  Abs/1 -> Compare To Threshold/1
  e/1 -> Product/1
  Logical Operator/1 -> Clamping/1  "Clamping"
  u/1 -> Product/2

== system ControlSystem/Variant system/SISO/Variant Controller/PID/Subsystem8/Clamping ==
  u : Inport
  antiw : Inport  Port=2
  e : Inport  Port=3
  Abs : Abs
  Compare To Threshold : simulink/Logic and Bit Operations/Compare To Constant  relop=>=  const=Threshold  OutDataTypeStr=boolean
  Compare To Zero : simulink/Logic and Bit Operations/Compare To Zero  relop=>=  OutDataTypeStr=boolean
  Logical Operator : Logic  OutDataTypeStr=boolean
  Product : Product
  Clamping : Outport
  wires:
  u/1 -> Product/2
  Logical Operator/1 -> Clamping/1  "Clamping"
  e/1 -> Product/1
  Abs/1 -> Compare To Threshold/1
  Product/1 -> Compare To Zero/1
  Compare To Threshold/1 -> Logical Operator/1
  Compare To Zero/1 -> Logical Operator/2
  antiw/1 -> Abs/1

== system ControlSystem/Variant system/SISO/Variant Controller/PID/Subsystem9/Clamping ==
  u : Inport
  antiw : Inport  Port=2
  e : Inport  Port=3
  Abs : Abs
  Compare To Threshold : simulink/Logic and Bit Operations/Compare To Constant  relop=>=  const=Threshold  OutDataTypeStr=boolean
  Compare To Zero : simulink/Logic and Bit Operations/Compare To Zero  relop=>=  OutDataTypeStr=boolean
  Logical Operator : Logic  OutDataTypeStr=boolean
  Product : Product
  Clamping : Outport
  wires:
  antiw/1 -> Abs/1
  Compare To Zero/1 -> Logical Operator/2
  Compare To Threshold/1 -> Logical Operator/1
  Product/1 -> Compare To Zero/1
  Abs/1 -> Compare To Threshold/1
  e/1 -> Product/1
  Logical Operator/1 -> Clamping/1  "Clamping"
  u/1 -> Product/2

== system ControlSystem/Variant system/SISO/Variant Controller/Rlocusantiwindup/Subsystem1/Clamping ==
  u : Inport
  antiw : Inport  Port=2
  e : Inport  Port=3
  Abs : Abs
  Compare To Threshold : simulink/Logic and Bit Operations/Compare To Constant  relop=>=  const=Threshold  OutDataTypeStr=boolean
  Compare To Zero : simulink/Logic and Bit Operations/Compare To Zero  relop=>=  OutDataTypeStr=boolean
  Logical Operator : Logic  OutDataTypeStr=boolean
  Product : Product
  Clamping : Outport
  wires:
  antiw/1 -> Abs/1
  Compare To Zero/1 -> Logical Operator/2
  Compare To Threshold/1 -> Logical Operator/1
  Product/1 -> Compare To Zero/1
  Abs/1 -> Compare To Threshold/1
  e/1 -> Product/1
  Logical Operator/1 -> Clamping/1  "Clamping"
  u/1 -> Product/2
